simulink model "stepResponse"  (R2021a)
settings: configuration reference "ctrlConfigSet" (kept outside this file)
undefined symbols (not defined in the file or in its folder): TFinal, uavParam
settings Model: DataDictionary=stepResponseData.sldd  SimulationMode=accelerator  Creator=The MathWorks, Inc.  LastModifiedBy=The MathWorks, Inc.
settings ConfigSetRef: SourceName=ctrlConfigSet

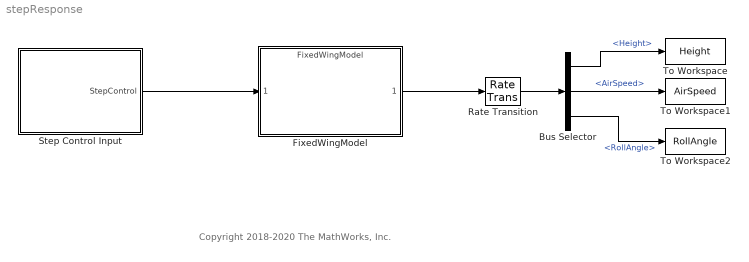
== system stepResponse ==
  note: Copyright 2018-2020 The MathWorks, Inc.
  Bus Selector : BusSelector  OutputSignals=Height,AirSpeed,RollAngle
  FixedWingModel : ModelReference  ModelNameDialog=FixedWingModel  SimulationMode=Normal  ModelReferenceVersion=1.27
  Rate Transition : RateTransition  OutPortSampleTime=0.1
  Step Control Input : Subsystem  Variant=on  VariantControlMode=label  LabelModeActiveChoice=StepRollAngle  mask{StepControl=RollAngle Step Control}
      mask prompts: StepControl "Step control mode:"
      mask init:
      | switch StepControl
      |     case 1
      |         set_param(gcb,'LabelModeActiveChoice', 'StepHeight');
      |     case 2
      |         set_param(gcb,'LabelModeActiveChoice', 'StepAirSpeed');
      |     case 3
      |         set_param(gcb,'LabelModeActiveChoice', 'StepRollAngle');
      | end
      mask TypeOptions StepControl: Height Step Control | AirSpeed Step Control | RollAngle Step Control
  To Workspace : ToWorkspace  VariableName=Height  SaveFormat=Timeseries  SampleTime=-1
  To Workspace1 : ToWorkspace  VariableName=AirSpeed  SaveFormat=Timeseries  SampleTime=-1
  To Workspace2 : ToWorkspace  VariableName=RollAngle  SaveFormat=Timeseries  SampleTime=-1
  wires:
  Bus Selector/1 -> To Workspace/1  "<Height>"
  Bus Selector/2 -> To Workspace1/1  "<AirSpeed>"
  Bus Selector/3 -> To Workspace2/1  "<RollAngle>"
  Step Control Input/1(StepControl) -> FixedWingModel/1
  FixedWingModel/1 -> Rate Transition/1
  Rate Transition/1 -> Bus Selector/1

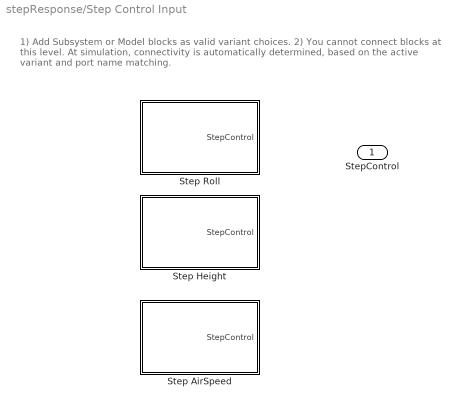
== system stepResponse/Step Control Input ==
  note: 1) Add Subsystem or Model blocks as valid variant choices.
      | 2) You cannot connect blocks at this level. At simulation, connectivity is automatically
      | determined, based on the active variant and port name matching.
  Step AirSpeed : Subsystem  VariantControl=StepAirSpeed
  Step Height : Subsystem  VariantControl=StepHeight
  Step Roll : Subsystem  VariantControl=StepRollAngle
  StepControl : Outport  VectorParamsAs1DForOutWhenUnconnected=off

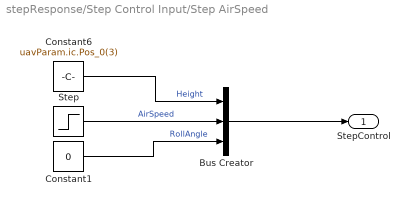
== system stepResponse/Step Control Input/Step AirSpeed ==
  Bus Creator : BusCreator  Inputs=3  OutDataTypeStr=Bus: FixedWingControlBus  NonVirtualBus=on
  Constant1 : Constant  Value=0
  Constant6 : Constant  Value=uavParam.ic.Pos_0(3)
  Step : Step  Time=TFinal/2  Before=18  After=19  SampleTime=0
  StepControl : Outport  VectorParamsAs1DForOutWhenUnconnected=off
  wires:
  Constant1/1 -> Bus Creator/3  "RollAngle"
  Constant6/1 -> Bus Creator/1  "Height"
  Step/1 -> Bus Creator/2  "AirSpeed"
  Bus Creator/1 -> StepControl/1

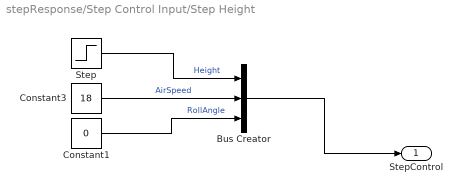
== system stepResponse/Step Control Input/Step Height ==
  Bus Creator : BusCreator  Inputs=3  OutDataTypeStr=Bus: FixedWingControlBus  NonVirtualBus=on
  Constant1 : Constant  Value=0
  Constant3 : Constant  Value=18
  Step : Step  Time=TFinal/2  Before=uavParam.ic.Pos_0(3)  After=uavParam.ic.Pos_0(3)+5  SampleTime=0
  StepControl : Outport  VectorParamsAs1DForOutWhenUnconnected=off
  wires:
  Bus Creator/1 -> StepControl/1
  Constant3/1 -> Bus Creator/2  "AirSpeed"
  Step/1 -> Bus Creator/1  "Height"
  Constant1/1 -> Bus Creator/3  "RollAngle"

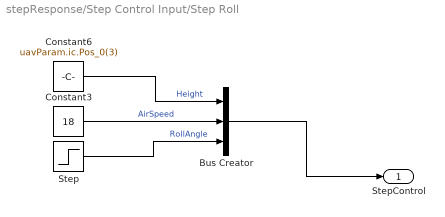
== system stepResponse/Step Control Input/Step Roll ==
  Bus Creator : BusCreator  Inputs=3  OutDataTypeStr=Bus: FixedWingControlBus  NonVirtualBus=on
  Constant3 : Constant  Value=18
  Constant6 : Constant  Value=uavParam.ic.Pos_0(3)
  Step : Step  Time=TFinal/2  After=pi/6  SampleTime=0
  StepControl : Outport  VectorParamsAs1DForOutWhenUnconnected=off
  wires:
  Step/1 -> Bus Creator/3  "RollAngle"
  Constant6/1 -> Bus Creator/1  "Height"
  Constant3/1 -> Bus Creator/2  "AirSpeed"
  Bus Creator/1 -> StepControl/1
